simulink model "TargetPosVel"  (R2025a)
settings: Solver=ode4  StartTime=0.0  StopTime=stopTime  FixedStep=timeStep  RelTol=1e-3
values from neighbouring files (symbols this model uses):
  rand_vec = [0, rand(), rand()]    [model_parameters.m]
undefined symbols (not defined in the file or in its folder): angular_rate_noise_ON, angular_rate_noise_power, c, CD, dayValue, dimx, dimz, hourValue, I, I_W, IAU, K_optics, kd, kq, max_h, max_t, minuteValue, mu_E, Omega_E, Phi, pointing_body, q, quat0, quaternion_bias, quaternion_noise_ON, quaternion_sigma, R_E, rcp, res_dipole, secondValue, sma, timeStep, w0, WMM2020, yearValue
libraries: aerolibutil x19, matrix_library x10, aerolibtransform2 x8, vrlib x5, simulink x1, sharedTrackingLibrary x1, aerolibatmos2 x1, aerolibgravity2 x1, sharedtransform x1, sensorgpslib x1, visionsources x1
(part 1 of 2)
settings Model: Creator=nicolasgagliardi  LastModifiedBy=ako

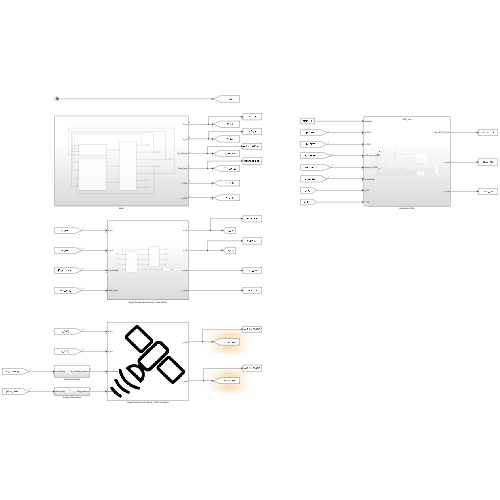
[thumbnail: Simulink's stored preview of the top-level diagram]
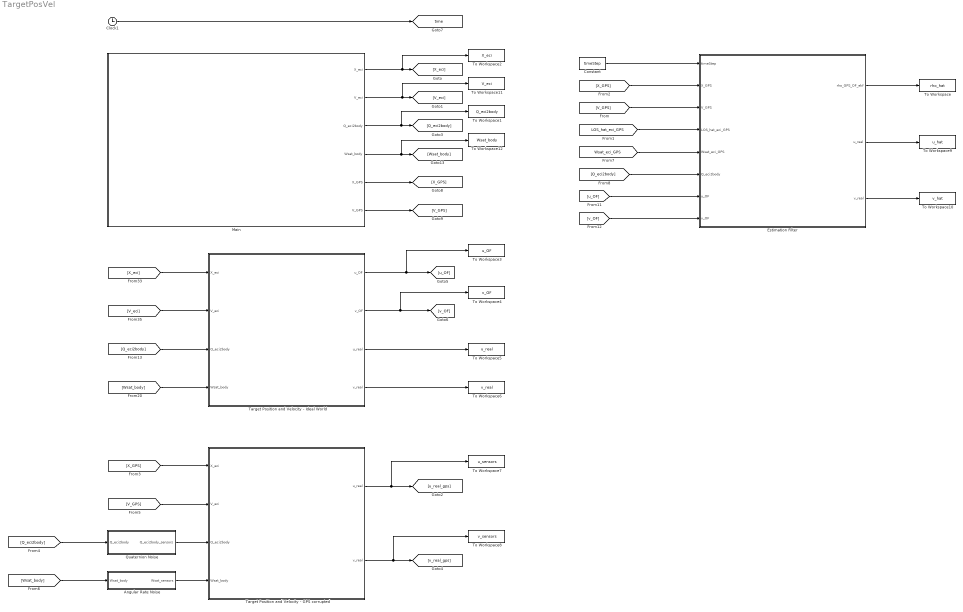
== system TargetPosVel ==
  Angular Rate Noise : Subsystem
  Clock1 : Clock
  Constant : Constant  Value=timeStep
  Estimation Filter : Subsystem  Variant=on  EmptyChoice=on
  Main : Subsystem
  Quaternion Noise : Subsystem
  Target Position and Velocity - GPS corrupted : Subsystem
      mask Display: image('gps.png');
  Target Position and Velocity - Ideal World : Subsystem
  To Workspace : ToWorkspace  VariableName=rho_hat  SaveFormat=Timeseries  SampleTime=-1
  To Workspace1 : ToWorkspace  VariableName=Q_eci2body  SaveFormat=Timeseries  SampleTime=-1
  To Workspace10 : ToWorkspace  VariableName=v_hat  SaveFormat=Timeseries  SampleTime=-1
  To Workspace11 : ToWorkspace  VariableName=V_eci  SaveFormat=Timeseries  SampleTime=-1
  To Workspace12 : ToWorkspace  VariableName=Wsat_body  SaveFormat=Timeseries  SampleTime=-1
  To Workspace2 : ToWorkspace  VariableName=X_eci  SaveFormat=Timeseries  SampleTime=-1
  To Workspace3 : ToWorkspace  VariableName=u_OF  SaveFormat=Timeseries  SampleTime=-1
  To Workspace4 : ToWorkspace  VariableName=v_OF  SaveFormat=Timeseries  SampleTime=-1
  To Workspace5 : ToWorkspace  VariableName=u_real  SaveFormat=Timeseries  SampleTime=-1
  To Workspace6 : ToWorkspace  VariableName=v_real  SaveFormat=Timeseries  SampleTime=-1
  To Workspace7 : ToWorkspace  VariableName=u_sensors  SaveFormat=Timeseries  SampleTime=-1
  To Workspace8 : ToWorkspace  VariableName=v_sensors  SaveFormat=Timeseries  SampleTime=-1
  To Workspace9 : ToWorkspace  VariableName=u_hat  SaveFormat=Timeseries  SampleTime=-1
  tag scope: time=global
  wires:
  [Q_eci2body] -> Target Position and Velocity - Ideal World/3(Q_eci2body)
  [Wsat_body] -> Target Position and Velocity - Ideal World/4(Wsat_body)
  Main/1(X_eci) -> [X_eci], To Workspace2/1
  Main/3(Q_eci2body) -> [Q_eci2body], To Workspace1/1
  Main/4(Wsat_body) -> To Workspace12/1, [Wsat_body]
  Main/2(V_eci) -> [V_eci], To Workspace11/1
  Target Position and Velocity - Ideal World/1(u_OF) -> To Workspace3/1, [u_OF]
  Main/5(X_GPS) -> [X_GPS]
  Main/6(V_GPS) -> [V_GPS]
  [V_eci] -> Target Position and Velocity - Ideal World/2(V_eci)
  Target Position and Velocity - GPS corrupted/1(u_real) -> [u_real_gps], To Workspace7/1
  Target Position and Velocity - GPS corrupted/2(v_real) -> [v_real_gps], To Workspace8/1
  [X_eci] -> Target Position and Velocity - Ideal World/1(X_eci)
  [X_GPS] -> Target Position and Velocity - GPS corrupted/1(X_eci)
  [V_GPS] -> Target Position and Velocity - GPS corrupted/2(V_eci)
  Target Position and Velocity - Ideal World/4(v_real) -> To Workspace6/1
  Target Position and Velocity - Ideal World/3(u_real) -> To Workspace5/1
  [Wsat_body] -> Angular Rate Noise/1(Wsat_body)
  Target Position and Velocity - Ideal World/2(v_OF) -> [v_OF], To Workspace4/1
  Clock1/1 -> [time]
  [Q_eci2body] -> Quaternion Noise/1(Q_eci2body)
  Quaternion Noise/1(Q_eci2body_sensors) -> Target Position and Velocity - GPS corrupted/3(Q_eci2body)
  Angular Rate Noise/1(Wsat_sensors) -> Target Position and Velocity - GPS corrupted/4(Wsat_body)
  Constant/1 -> Estimation Filter/1(timeStep)
  [X_GPS] -> Estimation Filter/2(X_GPS)
  [V_GPS] -> Estimation Filter/3(V_GPS)
  [LOS_hat_eci_GPS] -> Estimation Filter/4(LOS_hat_eci_GPS)
  [Wsat_eci_GPS] -> Estimation Filter/5(Wsat_eci_GPS)
  [Q_eci2body] -> Estimation Filter/6(Q_eci2body)
  [u_OF] -> Estimation Filter/7(u_OF)
  [v_OF] -> Estimation Filter/8(v_OF)
  Estimation Filter/1(rho_GPS_OF_ekf) -> To Workspace/1
  Estimation Filter/2(u_real) -> To Workspace9/1
  Estimation Filter/3(v_real) -> To Workspace10/1

== system TargetPosVel/Angular Rate Noise ==
  Wsat_body : Inport
  Add : Sum
  Band-Limited White Noise : simulink/Sources/Band-Limited White Noise  Cov=[angular_rate_noise_power]  Ts=timeStep  seed=[23341,23342,23343]
  Constant : Constant  Value=angular_rate_noise_ON
  Switch : Switch  Criteria=u2 ~= 0  SaturateOnIntegerOverflow=off  InputSameDT=off
  Wsat_sensors : Outport
  wires:
  Wsat_body/1 -> Switch/3, Add/2
  Add/1 -> Switch/1
  Constant/1 -> Switch/2
  Switch/1 -> Wsat_sensors/1
  Band-Limited White Noise/1 -> Add/1

== system TargetPosVel/Estimation Filter ==
  timeStep : Inport
  X_GPS : Inport  Port=2
  V_GPS : Inport  Port=3
  LOS_hat_eci_GPS : Inport  Port=4
  Wsat_eci_GPS : Inport  Port=5
  Q_eci2body : Inport  Port=6
  u_OF : Inport  Port=7
  v_OF : Inport  Port=8
  EKF_rho : Subsystem  VariantControl="estimation_filter == \"EKF_rho\""
  rho_GPS_OF_ekf : Outport
  u_real : Outport  Port=2
  v_real : Outport  Port=3

== system TargetPosVel/Main ==
  Attiude Controller : Subsystem  Variant=on  EmptyChoice=on
  Environmental Torques : Subsystem  Variant=on  EmptyChoice=on
  Spacecraft Dynamics : Subsystem
  X_eci : Outport
  V_eci : Outport  Port=2
  Q_eci2body : Outport  Port=3
  Wsat_body : Outport  Port=4
  X_GPS : Outport  Port=5
  V_GPS : Outport  Port=6
  wires:
  Spacecraft Dynamics/1(X_eci) -> Attiude Controller/1(r_ECI), Environmental Torques/1(X_eci), X_eci/1
  Spacecraft Dynamics/2(V_eci) -> Environmental Torques/2(V_eci), Attiude Controller/2(v_ECI), V_eci/1
  Spacecraft Dynamics/3(Q_eci2body) -> Environmental Torques/3(qECI2body), Attiude Controller/4(q_ECI2body), Q_eci2body/1
  Spacecraft Dynamics/4(W_sat_body) -> Attiude Controller/3(omega_b), Wsat_body/1
  Spacecraft Dynamics/6(X_GPS) -> X_GPS/1
  Spacecraft Dynamics/7(V_GPS) -> V_GPS/1
  Attiude Controller/1(h) -> Spacecraft Dynamics/2(h_rw)
  Attiude Controller/2(dh_dt) -> Spacecraft Dynamics/3(hdot_rw)
  Spacecraft Dynamics/5(t_JD) -> Environmental Torques/4(t_JD)
  Environmental Torques/1(T_env) -> Spacecraft Dynamics/1(T_env)

== system TargetPosVel/Quaternion Noise ==
  Q_eci2body : Inport
  Constant : Constant  Value=quaternion_noise_ON
  Constant1 : Constant  Value=quaternion_bias
  Constant2 : Constant  Value=quaternion_sigma
  MATLAB Function : MATLAB Function  TreatAsAtomicUnit=on
  Quaternion Multiplication : aerolibutil/Quaternion Multiplication
  Quaternion Multiplication2 : aerolibutil/Quaternion Multiplication
  Rotation Angles to Quaternions : Angle2Quat
      settings: AttributesFormatString=Rotation Order: %<rotationOrder>
  Rotation Angles to Quaternions1 : Angle2Quat
      settings: AttributesFormatString=Rotation Order: %<rotationOrder>
  Signal Specification : SignalSpecification  Dimensions=3
  Switch : Switch  Criteria=u2 ~= 0  SaturateOnIntegerOverflow=off  InputSameDT=off
  Q_eci2body_sensors : Outport
  wires:
  Q_eci2body/1 -> Quaternion Multiplication/2, Switch/3
  Rotation Angles to Quaternions/1 -> Quaternion Multiplication/1
  Switch/1 -> Q_eci2body_sensors/1
  Constant/1 -> Switch/2
  Constant1/1 -> Rotation Angles to Quaternions/1
  Constant2/1 -> MATLAB Function/1(quaternion_sigma)
  MATLAB Function/1(angle_noise) -> Signal Specification/1
  Quaternion Multiplication/1 -> Quaternion Multiplication2/2
  Quaternion Multiplication2/1 -> Switch/1
  Signal Specification/1 -> Rotation Angles to Quaternions1/1
  Rotation Angles to Quaternions1/1 -> Quaternion Multiplication2/1

== system TargetPosVel/Target Position and Velocity - GPS corrupted ==
  X_eci : Inport
  V_eci : Inport  Port=2
  Q_eci2body : Inport  Port=3
  Wsat_body : Inport  Port=4
  LLA conversion : Subsystem
  LOS Calculations : Subsystem
  Pixel shift : Subsystem
  To Workspace : ToWorkspace  VariableName=lla_tar_gps  SampleTime=-1
  u_real : Outport
  v_real : Outport  Port=2
  wires:
  LOS Calculations/3(Vtar_eci) -> Pixel shift/4(Vtar_eci)
  LOS Calculations/2(Rtar_eci) -> Pixel shift/3(Rtar_eci)
  LLA conversion/1(LLAtar) -> To Workspace/1
  LOS Calculations/4(Rtar_ecef) -> LLA conversion/1(Rtar_ecef)
  LOS Calculations/1(rho) -> Pixel shift/2(rho)
  Pixel shift/2(v_real) -> v_real/1
  Pixel shift/1(u_real) -> u_real/1
  Wsat_body/1 -> LOS Calculations/4(Wsat_b)
  X_eci/1 -> LOS Calculations/3(Rsat)
  V_eci/1 -> LOS Calculations/2(Vsat)
  Q_eci2body/1 -> LOS Calculations/1(Q_eci2body), Pixel shift/1(Q_eci2body)

== system TargetPosVel/Target Position and Velocity - Ideal World ==
  X_eci : Inport
  V_eci : Inport  Port=2
  Q_eci2body : Inport  Port=3
  Wsat_body : Inport  Port=4
  LLA conversion : Subsystem
  LOS Calculations : Subsystem
  Pixel shift : Subsystem
  To Workspace : ToWorkspace  VariableName=lla_tar  SampleTime=-1
  u_OF : Outport
  v_OF : Outport  Port=2
  u_real : Outport  Port=3
  v_real : Outport  Port=4
  wires:
  Q_eci2body/1 -> LOS Calculations/1(Q_eci2body), Pixel shift/1(Q_eci2body)
  V_eci/1 -> LOS Calculations/2(Vsat)
  X_eci/1 -> LOS Calculations/3(Rsat)
  Wsat_body/1 -> LOS Calculations/4(Wsat_b)
  Pixel shift/1(u_OF) -> u_OF/1
  Pixel shift/2(v_OF) -> v_OF/1
  LOS Calculations/1(rho) -> Pixel shift/2(rho)
  LOS Calculations/4(Rtar_ecef) -> LLA conversion/1(Rtar_ecef)
  LLA conversion/1(LLAtar) -> To Workspace/1
  LOS Calculations/2(Rtar_eci) -> Pixel shift/3(Rtar_eci)
  LOS Calculations/3(Vtar_eci) -> Pixel shift/4(Vtar_eci)
  Pixel shift/3(u_real) -> u_real/1
  Pixel shift/4(v_real) -> v_real/1

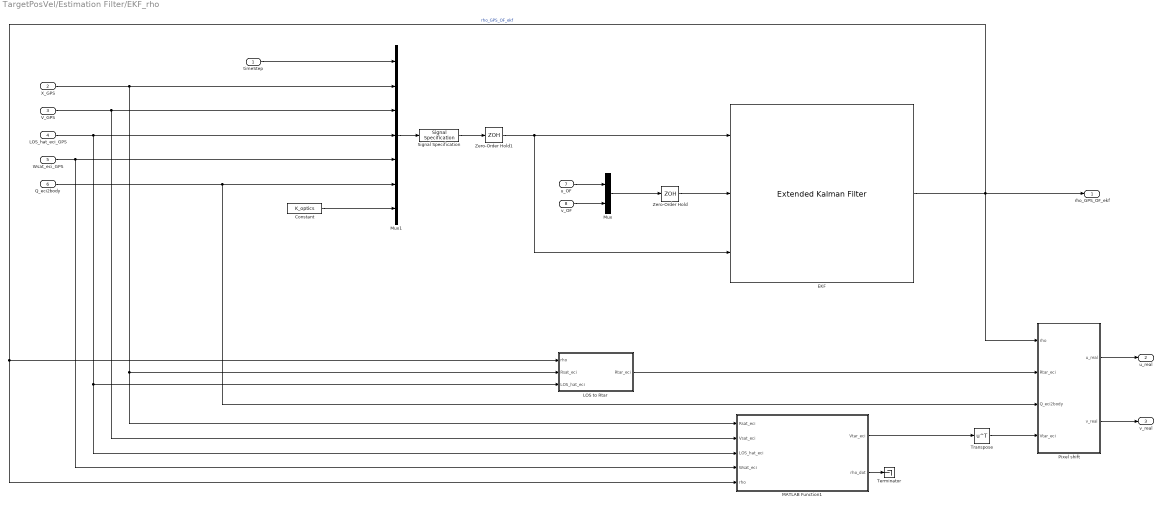
== system TargetPosVel/Estimation Filter/EKF_rho ==
  timeStep : Inport
  X_GPS : Inport  Port=2
  V_GPS : Inport  Port=3
  LOS_hat_eci_GPS : Inport  Port=4
  Wsat_eci_GPS : Inport  Port=5
  Q_eci2body : Inport  Port=6
  u_OF : Inport  Port=7
  v_OF : Inport  Port=8
  Constant : Constant  Value=K_optics
  EKF : sharedTrackingLibrary/Extended Kalman Filter  StateTransitionFcn=rhoSTF  HasStateTransitionJacobianFcn=off  HasAdditiveProcessNoise=Additive  ProcessNoise=Q  HasTimeVaryingProcessNoise=off  HasStateTransitionFcnExtraArgument=1  InitialState=rho_0  InitialStateCovariance=20  MeasurementFcn1=rhoMF  HasMeasurementJacobianFcn1=off  HasMeasurementEnablePort1=off  HasAdditiveMeasurementNoise1=Additive  MeasurementNoise1=[0.1,0;0,0.1]  HasTimeVaryingMeasurementNoise1=off  HasMeasurementFcnExtraArgument1=1  HasMeasurementWrapping1=off  MeasurementFcn2=myMeasurementFcn  HasMeasurementJacobianFcn2=off  HasMeasurementEnablePort2=off  HasAdditiveMeasurementNoise2=Additive  MeasurementNoise2=1  HasTimeVaryingMeasurementNoise2=off  HasMeasurementFcnExtraArgument2=0  HasMeasurementWrapping2=off  MeasurementFcn3=myMeasurementFcn  HasMeasurementJacobianFcn3=off  HasMeasurementEnablePort3=off  HasAdditiveMeasurementNoise3=Additive  MeasurementNoise3=1  HasTimeVaryingMeasurementNoise3=off  HasMeasurementFcnExtraArgument3=0  HasMeasurementWrapping3=off  MeasurementFcn4=myMeasurementFcn  HasMeasurementJacobianFcn4=off  HasMeasurementEnablePort4=off  HasAdditiveMeasurementNoise4=Additive  MeasurementNoise4=1  HasTimeVaryingMeasurementNoise4=off  HasMeasurementFcnExtraArgument4=0  HasMeasurementWrapping4=off  MeasurementFcn5=myMeasurementFcn  HasMeasurementJacobianFcn5=off  HasMeasurementEnablePort5=off  HasAdditiveMeasurementNoise5=Additive  MeasurementNoise5=1  HasTimeVaryingMeasurementNoise5=off  HasMeasurementFcnExtraArgument5=0  HasMeasurementWrapping5=off  EnableMultirate=off  StateTransitionFcnSampleTime=1  MeasurementFcn1SampleTime=1  MeasurementFcn2SampleTime=1  MeasurementFcn3SampleTime=1  MeasurementFcn4SampleTime=1  MeasurementFcn5SampleTime=1  UseCurrentEstimator=on  OutputStateCovariance=off  DataType=double  SampleTime=timeStep  NumberOfMeasurements=1
  LOS to Rtar : Subsystem
  MATLAB Function1 : MATLAB Function  TreatAsAtomicUnit=on
  Mux : Mux  Inputs=2
  Mux1 : Mux  Inputs=7
  Pixel shift : Subsystem
  Signal Specification : SignalSpecification  Dimensions=18
  Terminator : Terminator
  Transpose : Math  Operator=transpose
  Zero-Order Hold : ZeroOrderHold  SampleTime=timeStep
  Zero-Order Hold1 : ZeroOrderHold  SampleTime=timeStep
  rho_GPS_OF_ekf : Outport
  u_real : Outport  Port=2
  v_real : Outport  Port=3
  wires:
  timeStep/1 -> Mux1/1
  Mux1/1 -> Signal Specification/1
  Q_eci2body/1 -> Mux1/6, Pixel shift/3(Q_eci2body)
  Zero-Order Hold/1 -> EKF/2
  Zero-Order Hold1/1 -> EKF/1, EKF/3
  Mux/1 -> Zero-Order Hold/1
  Signal Specification/1 -> Zero-Order Hold1/1
  Wsat_eci_GPS/1 -> Mux1/5, MATLAB Function1/4(Wsat_eci)
  v_OF/1 -> Mux/2
  X_GPS/1 -> Mux1/2, MATLAB Function1/1(Rsat_eci), LOS to Rtar/2(Rsat_eci)
  LOS_hat_eci_GPS/1 -> Mux1/4, MATLAB Function1/3(LOS_hat_eci), LOS to Rtar/3(LOS_hat_eci)
  V_GPS/1 -> Mux1/3, MATLAB Function1/2(Vsat_eci)
  u_OF/1 -> Mux/1
  EKF/1 -> Pixel shift/1(rho), MATLAB Function1/5(rho), LOS to Rtar/1(rho), rho_GPS_OF_ekf/1  "rho_GPS_OF_ekf"
  Pixel shift/2(v_real) -> v_real/1
  Pixel shift/1(u_real) -> u_real/1
  MATLAB Function1/2(rho_dot) -> Terminator/1
  Constant/1 -> Mux1/7
  MATLAB Function1/1(Vtar_eci) -> Transpose/1
  Transpose/1 -> Pixel shift/4(Vtar_eci)
  LOS to Rtar/1(Rtar_eci) -> Pixel shift/2(Rtar_eci)

== system TargetPosVel/Main/Attiude Controller ==
  r_ECI : Inport
  v_ECI : Inport  Port=2
  omega_b : Inport  Port=3
  q_ECI2body : Inport  Port=4
  Controller OFF : Subsystem  VariantControl=controller_ON == 0
  Nadir Pointing Controller : Subsystem  VariantControl=controller_ON == 1
  h : Outport
  dh_dt : Outport  Port=2

== system TargetPosVel/Main/Environmental Torques ==
  X_eci : Inport
  V_eci : Inport  Port=2
  qECI2body : Inport  Port=3
  t_JD : Inport  Port=4
  Environmental Torques : Subsystem  VariantControl=env_torques_ON == 1
  Environmental Torques OFF : Subsystem  VariantControl=env_torques_ON == 0
  T_env : Outport

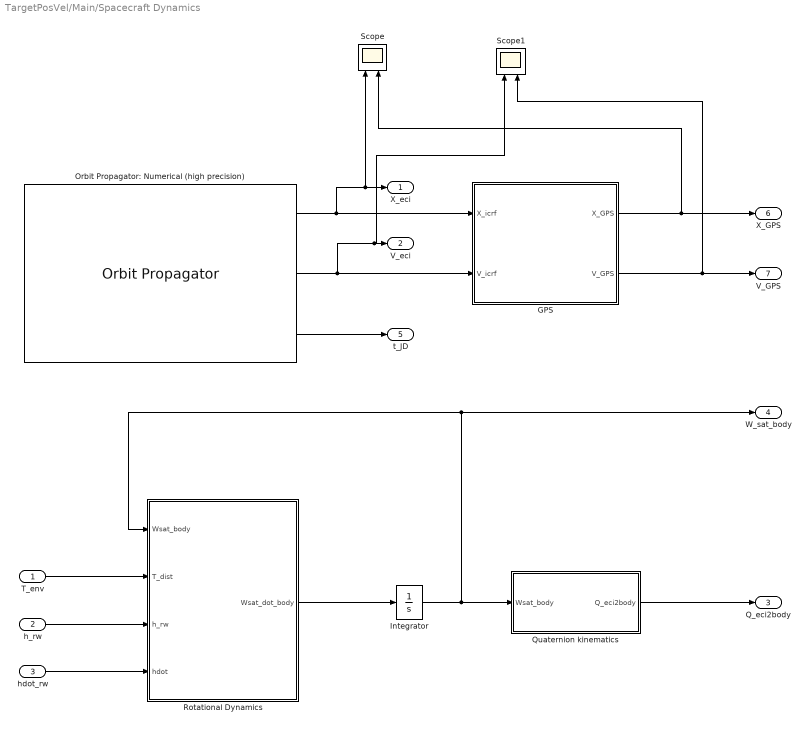
== system TargetPosVel/Main/Spacecraft Dynamics ==
  T_env : Inport
  h_rw : Inport  Port=2
  hdot_rw : Inport  Port=3
  GPS : Subsystem
  Integrator : Integrator  InitialCondition=w0
  Orbit Propagator: Numerical (high precision) : OrbitPropagator  propagator=Numerical (high precision)  startDate=jdate  mass=mass  action=None  semiMajorAxis=sma  eccentricity=ecc  inclination=inc_SSO  raan=RAAN  argPeriapsis=aop  trueAnomaly=truean  inertialPosition=[3649700.0 3308200.0 -4676600.0]  inertialVelocity=[-2750.8 6666.4 2573.4]  fixedPosition=[-4142689.0 -2676864.7 -4669861.6]  fixedVelocity=[1452.7 -6720.7 2568.1]  customR=3396200  customMu=4.305e13  customJ2=1.0826269e-03  customOmega=4.06125949e-3  F107ExtrapMethod=Least squares fit  MagneticIndexExtrapMethod=IGRF  dragCoeff=CD  dragArea=dimx*dimz  useEphemerisDateRange=off  ephemerisStartDate=jdate  ephemerisEndDate=jdate  includeSunGravity=off  reflectivityCoeff=q  srpArea=dimx*dimz
  Quaternion kinematics : Subsystem
  Rotational Dynamics : Subsystem
  Scope : Scope  NumInputPorts=2
      settings: ActiveDisplayYMinimum=-12780.9796153992  ActiveDisplayYMaximum=52179.154390941323
  Scope1 : Scope  NumInputPorts=2
      settings: ActiveDisplayYMinimum=-40.67155384373234  ActiveDisplayYMaximum=0.53047510275488818  DataLoggingVariableName=ScopeData4
  X_eci : Outport
  V_eci : Outport  Port=2
  Q_eci2body : Outport  Port=3
  W_sat_body : Outport  Port=4
  t_JD : Outport  Port=5
  X_GPS : Outport  Port=6
  V_GPS : Outport  Port=7
  wires:
  Orbit Propagator: Numerical (high precision)/3 -> t_JD/1
  Integrator/1 -> Quaternion kinematics/1(Wsat_body), W_sat_body/1, Rotational Dynamics/1(Wsat_body)
  GPS/1(X_GPS) -> X_GPS/1, Scope/2
  GPS/2(V_GPS) -> V_GPS/1, Scope1/2
  Orbit Propagator: Numerical (high precision)/1 -> GPS/1(X_icrf), X_eci/1, Scope/1
  T_env/1 -> Rotational Dynamics/2(T_dist)
  Rotational Dynamics/1(Wsat_dot_body) -> Integrator/1
  h_rw/1 -> Rotational Dynamics/3(h_rw)
  Orbit Propagator: Numerical (high precision)/2 -> Scope1/1, V_eci/1, GPS/2(V_icrf)
  hdot_rw/1 -> Rotational Dynamics/4(hdot)
  Quaternion kinematics/1(Q_eci2body) -> Q_eci2body/1

== system TargetPosVel/Target Position and Velocity - GPS corrupted/LLA conversion ==
  Rtar_ecef : Inport
  ECEF Position to LLA : ECEF2LLA
  Mux : Mux  Inputs=2
  LLAtar : Outport
  wires:
  Mux/1 -> LLAtar/1
  ECEF Position to LLA/2 -> Mux/2
  ECEF Position to LLA/1 -> Mux/1
  Rtar_ecef/1 -> ECEF Position to LLA/1

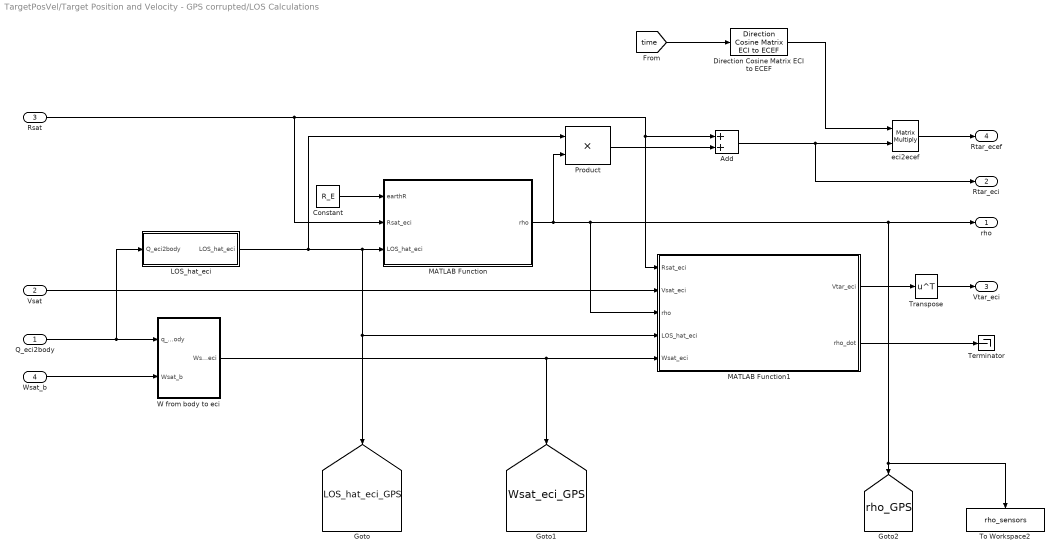
== system TargetPosVel/Target Position and Velocity - GPS corrupted/LOS Calculations ==
  Q_eci2body : Inport
  Vsat : Inport  Port=2
  Rsat : Inport  Port=3
  Wsat_b : Inport  Port=4
  Add : Sum
  Constant : Constant  Value=R_E
  Direction Cosine Matrix ECI to ECEF : aerolibtransform2/Direction Cosine Matrix ECI to ECEF  red=IAU-2000/2006  year=yearValue  month=January  day=1  hour=hourValue  min=minuteValue  sec=secondValue  deltaT=Sec  errorflag=Error  extraparamflag=off
      settings: AttributesFormatString=%<red>
  LOS_hat_eci : Subsystem
  MATLAB Function : MATLAB Function  TreatAsAtomicUnit=on
  MATLAB Function1 : MATLAB Function  TreatAsAtomicUnit=on
  Product : Product
  Terminator : Terminator
  To Workspace2 : ToWorkspace  VariableName=rho_sensors  SaveFormat=Timeseries  SampleTime=-1
  Transpose : Math  Operator=transpose
  "W from body to eci " : Subsystem
  eci2ecef : Product  Multiplication=Matrix(*)
  rho : Outport
  Rtar_eci : Outport  Port=2
  Vtar_eci : Outport  Port=3
  Rtar_ecef : Outport  Port=4
  tag scope: LOS_hat_eci_GPS=global, Wsat_eci_GPS=global, rho_GPS=global
  wires:
  eci2ecef/1 -> Rtar_ecef/1
  Add/1 -> Rtar_eci/1, eci2ecef/2
  Direction Cosine Matrix ECI to ECEF/1 -> eci2ecef/1
  Vsat/1 -> MATLAB Function1/2(Vsat_eci)
  LOS_hat_eci/1(LOS_hat_eci) -> Product/1, MATLAB Function/3(LOS_hat_eci), MATLAB Function1/4(LOS_hat_eci), [LOS_hat_eci_GPS]
  "W from body to eci "/1(Wsat_eci) -> [Wsat_eci_GPS], MATLAB Function1/5(Wsat_eci)
  Constant/1 -> MATLAB Function/1(earthR)
  Wsat_b/1 -> "W from body to eci "/2(Wsat_b)
  Rsat/1 -> MATLAB Function/2(Rsat_eci), Add/1, MATLAB Function1/1(Rsat_eci)
  MATLAB Function/1(rho) -> Product/2, MATLAB Function1/3(rho), rho/1, To Workspace2/1, [rho_GPS]
  Q_eci2body/1 -> "W from body to eci "/1(q_eci2body), LOS_hat_eci/1(Q_eci2body)
  Product/1 -> Add/2
  MATLAB Function1/2(rho_dot) -> Terminator/1
  MATLAB Function1/1(Vtar_eci) -> Transpose/1
  Transpose/1 -> Vtar_eci/1
  [time] -> Direction Cosine Matrix ECI to ECEF/1

== system TargetPosVel/Target Position and Velocity - GPS corrupted/Pixel shift ==
  Q_eci2body : Inport
  rho : Inport  Port=2
  Rtar_eci : Inport  Port=3
  Vtar_eci : Inport  Port=4
  Constant : Constant  Value=[0;0;Omega_E]
  Selector2 : Selector  InputPortWidth=3  IndexOptions=Index vector (dialog)  Indices=[1 2]  OutputSizes=1
  UV calculation : Subsystem
  Vim_body : Subsystem
  Vim_eci : Subsystem
  u_real : Outport
  v_real : Outport  Port=2
  wires:
  Constant/1 -> Vim_eci/3(We_eci)
  UV calculation/2(v_real) -> v_real/1
  UV calculation/1(u_real) -> u_real/1
  Vim_eci/1(Vim_eci) -> Vim_body/2(vec)
  Vim_body/1(vec_rot) -> Selector2/1
  rho/1 -> UV calculation/2(rho)
  Vtar_eci/1 -> Vim_eci/2(Vtar_eci)
  Q_eci2body/1 -> Vim_body/1(q)
  Selector2/1 -> UV calculation/1(Vim_body)
  Rtar_eci/1 -> Vim_eci/1(Rtar_eci)

== system TargetPosVel/Target Position and Velocity - Ideal World/LLA conversion ==
  Rtar_ecef : Inport
  ECEF Position to LLA : ECEF2LLA
  Mux : Mux  Inputs=2
  LLAtar : Outport
  wires:
  Rtar_ecef/1 -> ECEF Position to LLA/1
  ECEF Position to LLA/1 -> Mux/1
  ECEF Position to LLA/2 -> Mux/2
  Mux/1 -> LLAtar/1

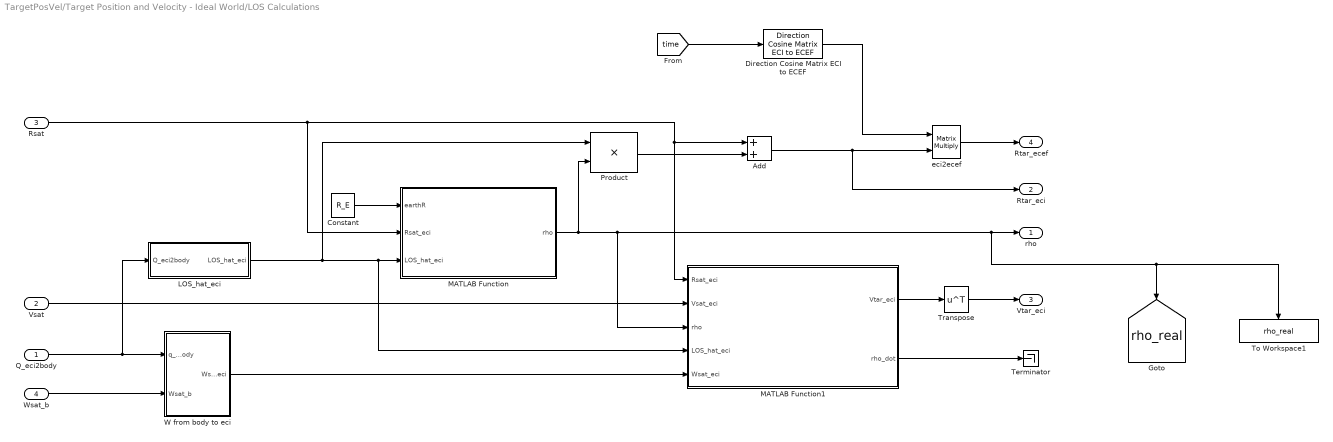
== system TargetPosVel/Target Position and Velocity - Ideal World/LOS Calculations ==
  Q_eci2body : Inport
  Vsat : Inport  Port=2
  Rsat : Inport  Port=3
  Wsat_b : Inport  Port=4
  Add : Sum
  Constant : Constant  Value=R_E
  Direction Cosine Matrix ECI to ECEF : aerolibtransform2/Direction Cosine Matrix ECI to ECEF  red=IAU-2000/2006  year=yearValue  month=January  day=1  hour=hourValue  min=minuteValue  sec=secondValue  deltaT=Sec  errorflag=Error  extraparamflag=off
      settings: AttributesFormatString=%<red>
  LOS_hat_eci : Subsystem
  MATLAB Function : MATLAB Function  TreatAsAtomicUnit=on
  MATLAB Function1 : MATLAB Function  TreatAsAtomicUnit=on
  Product : Product
  Terminator : Terminator
  To Workspace1 : ToWorkspace  VariableName=rho_real  SaveFormat=Timeseries  SampleTime=-1
  Transpose : Math  Operator=transpose
  "W from body to eci " : Subsystem
  eci2ecef : Product  Multiplication=Matrix(*)
  rho : Outport
  Rtar_eci : Outport  Port=2
  Vtar_eci : Outport  Port=3
  Rtar_ecef : Outport  Port=4
  tag scope: rho_real=global
  wires:
  Product/1 -> Add/2
  Q_eci2body/1 -> LOS_hat_eci/1(Q_eci2body), "W from body to eci "/1(q_eci2body)
  MATLAB Function/1(rho) -> [rho_real], To Workspace1/1, rho/1, MATLAB Function1/3(rho), Product/2
  Rsat/1 -> MATLAB Function1/1(Rsat_eci), Add/1, MATLAB Function/2(Rsat_eci)
  Wsat_b/1 -> "W from body to eci "/2(Wsat_b)
  Constant/1 -> MATLAB Function/1(earthR)
  "W from body to eci "/1(Wsat_eci) -> MATLAB Function1/5(Wsat_eci)
  LOS_hat_eci/1(LOS_hat_eci) -> MATLAB Function1/4(LOS_hat_eci), MATLAB Function/3(LOS_hat_eci), Product/1
  Vsat/1 -> MATLAB Function1/2(Vsat_eci)
  Direction Cosine Matrix ECI to ECEF/1 -> eci2ecef/1
  Add/1 -> eci2ecef/2, Rtar_eci/1
  eci2ecef/1 -> Rtar_ecef/1
  MATLAB Function1/2(rho_dot) -> Terminator/1
  MATLAB Function1/1(Vtar_eci) -> Transpose/1
  Transpose/1 -> Vtar_eci/1
  [time] -> Direction Cosine Matrix ECI to ECEF/1

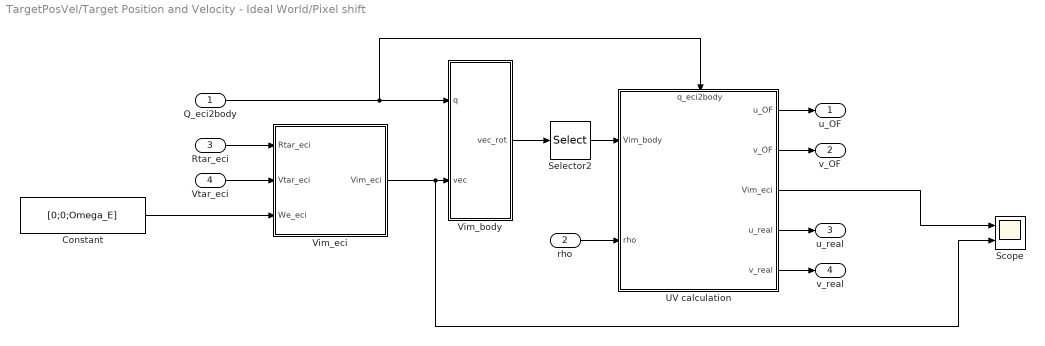
== system TargetPosVel/Target Position and Velocity - Ideal World/Pixel shift ==
  Q_eci2body : Inport
  rho : Inport  Port=2
  Rtar_eci : Inport  Port=3
  Vtar_eci : Inport  Port=4
  Constant : Constant  Value=[0;0;Omega_E]
  Scope : Scope  NumInputPorts=2
      settings: ActiveDisplayYMinimum=7345.085472920141  ActiveDisplayYMaximum=7801.8686248677177  DataLoggingVariableName=ScopeData5
  Selector2 : Selector  InputPortWidth=3  IndexOptions=Index vector (dialog)  Indices=[1 2]  OutputSizes=1
  UV calculation : Subsystem
      settings: PortSchema="{\"entries\":[{\"content\":{\"sides\":[{\"content\":{\"connectorIds\":[\"In1\",\"In2\"]},\"type\":\"ConnectorPlacement.EquallySpacedRectSide\",\"uuid\":\"7d962072-08bb-43f9-8096-b084f9aeb233\"},{\"content\":{\"connectorIds\":[\"Out1\",\"Out2\",\"Out3\",\"Out4\",\"Out5\"],\"side\":\"RIGHT\"},\"type\":\"ConnectorPlacement.EquallySpacedRectSide\",\"uuid\":\"b4a50fa6-2234-460e-9b12-c6b5a2f30818\"},{\"content\":{\"connectorIds\":[\"In3\"],\"side\":\"TOP\"},\"type\":\"ConnectorPlacement.EquallySpacedRectSide\",\"uuid\":\"25b05795-271b-402f-b612-88591474e4ef\"}]},\"type\":\"ConnectorPlacement.EquallySpacedConnector\",\"uuid\":\"2e7139ee-cebd-46fb-9053-110263a5a01d\"}],\"packageUris\":[\"http://schema.mathworks.com/mf0/Connector/R2020b\"],\"version\":\"1.0\"}"
  Vim_body : Subsystem
  Vim_eci : Subsystem
  u_OF : Outport
  v_OF : Outport  Port=2
  u_real : Outport  Port=3
  v_real : Outport  Port=4
  wires:
  Rtar_eci/1 -> Vim_eci/1(Rtar_eci)
  Selector2/1 -> UV calculation/1(Vim_body)
  Q_eci2body/1 -> Vim_body/1(q), UV calculation/3(q_eci2body)
  Vtar_eci/1 -> Vim_eci/2(Vtar_eci)
  rho/1 -> UV calculation/2(rho)
  Vim_body/1(vec_rot) -> Selector2/1
  Vim_eci/1(Vim_eci) -> Scope/2, Vim_body/2(vec)
  UV calculation/1(u_OF) -> u_OF/1
  UV calculation/2(v_OF) -> v_OF/1
  Constant/1 -> Vim_eci/3(We_eci)
  UV calculation/3(Vim_eci) -> Scope/1
  UV calculation/4(u_real) -> u_real/1
  UV calculation/5(v_real) -> v_real/1

== system TargetPosVel/Estimation Filter/EKF_rho/LOS to Rtar ==
  rho : Inport
  Rsat_eci : Inport  Port=2
  LOS_hat_eci : Inport  Port=3
  Add : Sum
  Product : Product
  Rtar_eci : Outport
  wires:
  LOS_hat_eci/1 -> Product/1
  rho/1 -> Product/2
  Product/1 -> Add/1
  Rsat_eci/1 -> Add/2
  Add/1 -> Rtar_eci/1

== system TargetPosVel/Estimation Filter/EKF_rho/Pixel shift ==
  rho : Inport
  Rtar_eci : Inport  Port=2
  Q_eci2body : Inport  Port=3
  Vtar_eci : Inport  Port=4
  Constant : Constant  Value=[0;0;Omega_E]
  Selector2 : Selector  InputPortWidth=3  IndexOptions=Index vector (dialog)  Indices=[1 2]  OutputSizes=1
  UV calculation : Subsystem
  Vim_body : Subsystem
  Vim_eci : Subsystem
  u_real : Outport
  v_real : Outport  Port=2
  wires:
  Constant/1 -> Vim_eci/3(We_eci)
  UV calculation/2(v_real) -> v_real/1
  UV calculation/1(u_real) -> u_real/1
  Vim_body/1(vec_rot) -> Selector2/1
  rho/1 -> UV calculation/2(rho)
  Vtar_eci/1 -> Vim_eci/2(Vtar_eci)
  Q_eci2body/1 -> Vim_body/1(q)
  Selector2/1 -> UV calculation/1(Vim_body)
  Rtar_eci/1 -> Vim_eci/1(Rtar_eci)
  Vim_eci/1(Vim_eci) -> Vim_body/2(vec)

== system TargetPosVel/Main/Attiude Controller/Controller OFF ==
  Constant : Constant  Value=0
  Constant1 : Constant  Value=0
  h : Outport
  dh_dt : Outport  Port=2
  wires:
  Constant/1 -> h/1
  Constant1/1 -> dh_dt/1

== system TargetPosVel/Main/Attiude Controller/Nadir Pointing Controller ==
  r_ECI : Inport
  v_ECI : Inport  Port=2
  omega_b : Inport  Port=3
  q_ECI2body : Inport  Port=4
  Nadir Pointing : Subsystem  TreatAsAtomicUnit=on
  Nadir pointing : Subsystem
  RW Saturation : Subsystem
  h : Outport
  dh_dt : Outport  Port=2
  wires:
  omega_b/1 -> Nadir pointing/2(omega_b), RW Saturation/2(omega)
  RW Saturation/2(dh_dt) -> dh_dt/1
  RW Saturation/1(h) -> h/1
  Nadir pointing/1(g) -> RW Saturation/1(g)
  Nadir Pointing/1(q_Err) -> Nadir pointing/1(qErr)
  Nadir Pointing/2(w_des) -> Nadir pointing/3(omega_des_b)
  r_ECI/1 -> Nadir Pointing/1(r_ECI)
  v_ECI/1 -> Nadir Pointing/2(v_ECI)
  q_ECI2body/1 -> Nadir Pointing/3(q_ECI2body)

== system TargetPosVel/Main/Environmental Torques/Environmental Torques ==
  X_eci : Inport
  V_eci : Inport  Port=2
  qECI2body : Inport  Port=3
  t_JD : Inport  Port=4
  Add : Sum  Inputs=++++
  "Aerodynamic Torque  " : Subsystem
  Gravity Gradient Torque : Subsystem
  Magnetic Torque : Subsystem
  Quaternions to Direction Cosine Matrix : sharedtransform/Quaternions to  Direction Cosine Matrix  aMode=aMode
  Solar Radiation Pressure Torque : Subsystem
  T_env : Outport
  wires:
  "Aerodynamic Torque  "/1(Tdrag) -> Add/2
  Quaternions to Direction Cosine Matrix/1 -> Magnetic Torque/2(DCM_eci2body), Solar Radiation Pressure Torque/1(DCM_eci2body), "Aerodynamic Torque  "/2(DCM_eci2body), Gravity Gradient Torque/1(DCM_eci2body)
  Gravity Gradient Torque/1(Tgg) -> Add/1
  X_eci/1 -> Solar Radiation Pressure Torque/2(X_eci), Magnetic Torque/1(X_eci), "Aerodynamic Torque  "/1(X_eci), Gravity Gradient Torque/2(X_eci)
  V_eci/1 -> "Aerodynamic Torque  "/3(V_eci)
  Solar Radiation Pressure Torque/1(T_srp) -> Add/3
  qECI2body/1 -> Quaternions to Direction Cosine Matrix/1
  t_JD/1 -> Solar Radiation Pressure Torque/3(t_JD)
  Magnetic Torque/1(Tmag) -> Add/4
  Add/1 -> T_env/1

== system TargetPosVel/Main/Environmental Torques/Environmental Torques OFF ==
  Constant : Constant  Value=0
  T_env : Outport
  wires:
  Constant/1 -> T_env/1

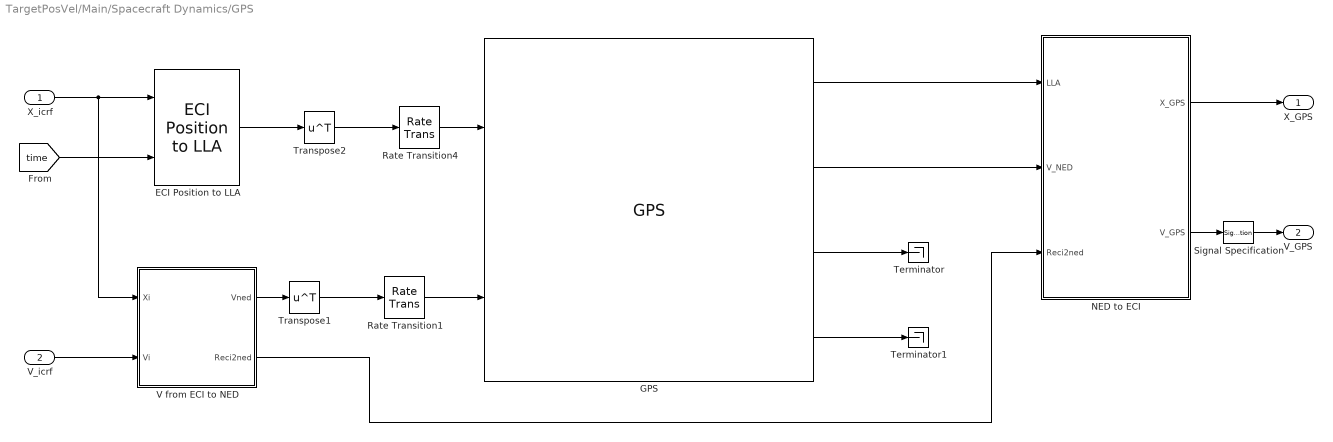
== system TargetPosVel/Main/Spacecraft Dynamics/GPS ==
  X_icrf : Inport
  V_icrf : Inport  Port=2
  ECI Position to LLA : aerolibtransform2/ECI Position to LLA  red=IAU-2000/2006  year=yearValue  month=January  day=1  hour=hourValue  min=minuteValue  sec=secondValue  deltaT=Sec  errorflag=Error  extraparamflag=off  eunits=Metric (MKS)  earthmodel=WGS84  flat=1/298.257223563  eqradius=6378137
      settings: AttributesFormatString=%<red>
  GPS : sensorgpslib/GPS  DispRefFrame=NED  PositionInputFormat=Geodetic  ReferenceLocation=[ 0, 0, 0 ]  HorizontalPositionAccuracy=GPSHAccuracy  VerticalPositionAccuracy=GPSVAccuracy  VelocityAccuracy=GPSVelAccuracy  DecayFactor=0  SeedDouble=67  SimulateUsing=Interpreted execution
  NED to ECI : Subsystem
  Rate Transition1 : RateTransition  OutPortSampleTime=timeStep
  Rate Transition4 : RateTransition  OutPortSampleTime=timeStep
  Signal Specification : SignalSpecification  Dimensions=3
  Terminator : Terminator
  Terminator1 : Terminator
  Transpose1 : Math  Operator=transpose
  Transpose2 : Math  Operator=transpose
  V from ECI to NED : Subsystem
  X_GPS : Outport
  V_GPS : Outport  Port=2
  wires:
  V_icrf/1 -> V from ECI to NED/2(Vi)
  ECI Position to LLA/1 -> Transpose2/1
  Rate Transition4/1 -> GPS/1
  Rate Transition1/1 -> GPS/2
  Transpose1/1 -> Rate Transition1/1
  Transpose2/1 -> Rate Transition4/1
  X_icrf/1 -> ECI Position to LLA/1, V from ECI to NED/1(Xi)
  GPS/3 -> Terminator/1
  GPS/4 -> Terminator1/1
  GPS/1 -> NED to ECI/1(LLA)
  GPS/2 -> NED to ECI/2(V_NED)
  NED to ECI/1(X_GPS) -> X_GPS/1
  V from ECI to NED/2(Reci2ned) -> NED to ECI/3(Reci2ned)
  V from ECI to NED/1(Vned) -> Transpose1/1
  [time] -> ECI Position to LLA/2
  Signal Specification/1 -> V_GPS/1
  NED to ECI/2(V_GPS) -> Signal Specification/1

== system TargetPosVel/Main/Spacecraft Dynamics/Quaternion kinematics ==
  Wsat_body : Inport
  Gain1 : Gain  Gain=0.5
  Integrator1 : Integrator  InitialCondition=quat0
  MATLAB Function : MATLAB Function  TreatAsAtomicUnit=on
  Product : Product  Multiplication=Matrix(*)
  Q_eci2body : Outport
  wires:
  Gain1/1 -> Product/1
  Wsat_body/1 -> MATLAB Function/1(omega)
  MATLAB Function/1(OMEGA) -> Gain1/1
  Integrator1/1 -> Q_eci2body/1, Product/2
  Product/1 -> Integrator1/1

== system TargetPosVel/Main/Spacecraft Dynamics/Rotational Dynamics ==
  Wsat_body : Inport
  T_dist : Inport  Port=2
  h_rw : Inport  Port=3
  hdot : Inport  Port=4
  Constant : Constant  Value=I
  Cross Product : matrix_library/Cross Product
  Invert 3x3 Matrix : aerolibutil/Invert  3x3 Matrix
  MatrixMultiply : Product  Multiplication=Matrix(*)
  MatrixMultiply1 : Product  Multiplication=Matrix(*)
  Minus : Sum  Inputs=+--
  Minus1 : Sum
  Wsat_dot_body : Outport
  wires:
  Invert 3x3 Matrix/1 -> MatrixMultiply1/1
  T_dist/1 -> Minus/1
  Minus1/1 -> Cross Product/2
  MatrixMultiply1/1 -> Wsat_dot_body/1
  Minus/1 -> MatrixMultiply1/2
  Constant/1 -> Invert 3x3 Matrix/1, MatrixMultiply/1
  Wsat_body/1 -> Cross Product/1, MatrixMultiply/2
  MatrixMultiply/1 -> Minus1/1
  Cross Product/1 -> Minus/2
  h_rw/1 -> Minus1/2
  hdot/1 -> Minus/3

== system TargetPosVel/Target Position and Velocity - GPS corrupted/LOS Calculations/LOS_hat_eci ==
  Q_eci2body : Inport
  Constant : Constant  Value=pointing_body
  Quaternion Inverse : aerolibutil/Quaternion Inverse
  Quaternion Rotation : aerolibutil/Quaternion Rotation
  LOS_hat_eci : Outport
  wires:
  Quaternion Rotation/1 -> LOS_hat_eci/1  "LOS_hat_eci"
  Constant/1 -> Quaternion Rotation/2
  Quaternion Inverse/1 -> Quaternion Rotation/1  "q_body2eci"
  Q_eci2body/1 -> Quaternion Inverse/1

== system TargetPosVel/Target Position and Velocity - GPS corrupted/LOS Calculations/W from body to eci  ==
  q_eci2body : Inport
  Wsat_b : Inport  Port=2
  Quaternion Inverse : aerolibutil/Quaternion Inverse
  Quaternion Rotation : aerolibutil/Quaternion Rotation
  Wsat_eci : Outport
  wires:
  Quaternion Rotation/1 -> Wsat_eci/1
  Wsat_b/1 -> Quaternion Rotation/2
  q_eci2body/1 -> Quaternion Inverse/1
  Quaternion Inverse/1 -> Quaternion Rotation/1

== system TargetPosVel/Target Position and Velocity - GPS corrupted/Pixel shift/UV calculation ==
  Vim_body : Inport
  rho : Inport  Port=2
  True shift : Subsystem
  u_real : Outport
  v_real : Outport  Port=2
  wires:
  rho/1 -> True shift/2(rho)
  Vim_body/1 -> True shift/1(Vim_body)
  True shift/2(v) -> v_real/1
  True shift/1(u) -> u_real/1

== system TargetPosVel/Target Position and Velocity - GPS corrupted/Pixel shift/Vim_body ==
  q : Inport
  vec : Inport  Port=2
  Quaternion Rotation : aerolibutil/Quaternion Rotation
  vec_rot : Outport
  wires:
  Quaternion Rotation/1 -> vec_rot/1
  vec/1 -> Quaternion Rotation/2
  q/1 -> Quaternion Rotation/1

== system TargetPosVel/Target Position and Velocity - GPS corrupted/Pixel shift/Vim_eci ==
  Rtar_eci : Inport
  Vtar_eci : Inport  Port=2
  We_eci : Inport  Port=3
  Cross Product : matrix_library/Cross Product
  Subtract : Sum  Inputs=+-
  Vim_eci : Outport
  wires:
  Vtar_eci/1 -> Subtract/1
  Subtract/1 -> Vim_eci/1
  Cross Product/1 -> Subtract/2
  Rtar_eci/1 -> Cross Product/2
  We_eci/1 -> Cross Product/1

== system TargetPosVel/Target Position and Velocity - Ideal World/LOS Calculations/LOS_hat_eci ==
  Q_eci2body : Inport
  Constant : Constant  Value=pointing_body
  Quaternion Inverse : aerolibutil/Quaternion Inverse
  Quaternion Rotation : aerolibutil/Quaternion Rotation
  LOS_hat_eci : Outport
  wires:
  Q_eci2body/1 -> Quaternion Inverse/1
  Quaternion Inverse/1 -> Quaternion Rotation/1  "q_body2eci"
  Constant/1 -> Quaternion Rotation/2
  Quaternion Rotation/1 -> LOS_hat_eci/1  "LOS_hat_eci"

== system TargetPosVel/Target Position and Velocity - Ideal World/LOS Calculations/W from body to eci  ==
  q_eci2body : Inport
  Wsat_b : Inport  Port=2
  Quaternion Inverse : aerolibutil/Quaternion Inverse
  Quaternion Rotation : aerolibutil/Quaternion Rotation
  Wsat_eci : Outport
  wires:
  Quaternion Inverse/1 -> Quaternion Rotation/1
  q_eci2body/1 -> Quaternion Inverse/1
  Wsat_b/1 -> Quaternion Rotation/2
  Quaternion Rotation/1 -> Wsat_eci/1

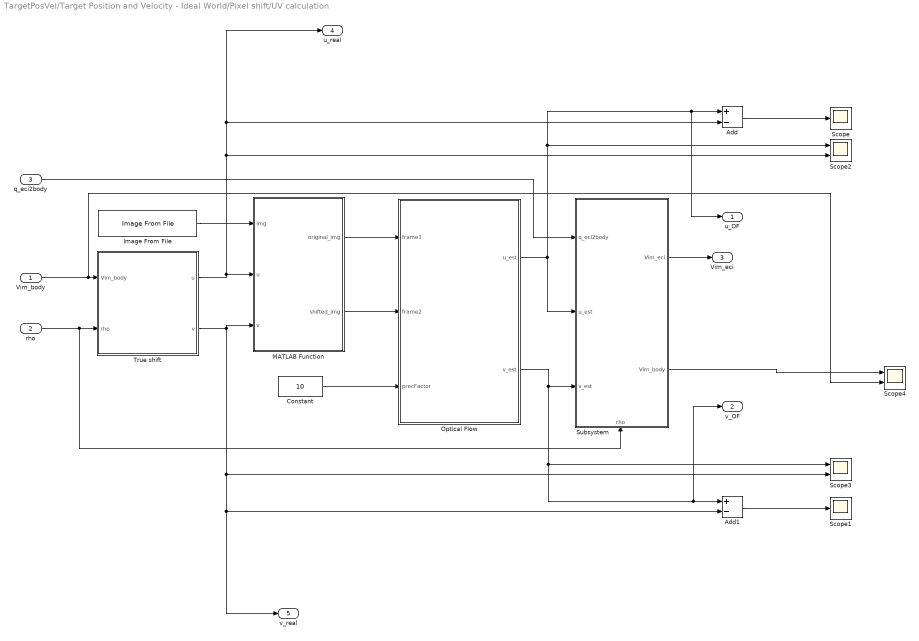
== system TargetPosVel/Target Position and Velocity - Ideal World/Pixel shift/UV calculation ==
  Vim_body : Inport
  rho : Inport  Port=2
  q_eci2body : Inport  Port=3
  Add : Sum  Inputs=+-
  Add1 : Sum  Inputs=+-
  Constant : Constant  Value=10
  Image From File : visionsources/Image From File  Tag=vipblks_nd  FileName=frame.jpg  Ts=inf  imagePorts=One multidimensional signal  OutPortLabels=R|G|B  ImageDataType=Inherit from input image  sdImageDataType=uint(8)  Signed=on  WordLength=16  FractionLengthMode=User-defined  FractionLength=15
  MATLAB Function : MATLAB Function  TreatAsAtomicUnit=on
  Optical Flow : MATLAB Function  TreatAsAtomicUnit=on
  Scope : Scope
      settings: Title=b_u  ActiveDisplayYMinimum=-0.079232845104481253  ActiveDisplayYMaximum=0.13207919106866894
  Scope1 : Scope
      settings: Title=b_v  ActiveDisplayYMinimum=-0.070013971574010736  ActiveDisplayYMaximum=0.11209756833780884  DataLoggingVariableName=ScopeData3
  Scope2 : Scope  NumInputPorts=2
      settings: Title=u vs u_est  ActiveDisplayYMinimum=-32.563714050832083  ActiveDisplayYMaximum=-30.048476216574212
  Scope3 : Scope  NumInputPorts=2
      settings: Title=v vs v_est  ActiveDisplayYMinimum=1.7373438554253244  ActiveDisplayYMaximum=2.0291840160638528  DataLoggingVariableName=ScopeData2
  Scope4 : Scope  NumInputPorts=2
      settings: ActiveDisplayYMinimum=-1  ActiveDisplayYMaximum=1  DataLoggingVariableName=ScopeData6
  Subsystem : Subsystem
      settings: PortSchema="{\"entries\":[{\"content\":{\"sides\":[{\"content\":{\"connectorIds\":[\"In1\",\"In2\",\"In3\"]},\"type\":\"ConnectorPlacement.EquallySpacedRectSide\",\"uuid\":\"00ab2d78-b092-482a-93cf-ae19a1715d5e\"},{\"content\":{\"connectorIds\":[\"Out1\",\"Out2\"],\"side\":\"RIGHT\"},\"type\":\"ConnectorPlacement.EquallySpacedRectSide\",\"uuid\":\"61835ddc-2b31-4e43-8d4a-874cf6b152c0\"},{\"content\":{\"side\":\"TOP\"},\"type\":\"ConnectorPlacement.EquallySpacedRectSide\",\"uuid\":\"ce3dab25-97d8-4e4a-ae1c-056d1a385cfa\"},{\"content\":{\"connectorIds\":[\"In4\"],\"side\":\"BOTTOM\"},\"type\":\"ConnectorPlacement.EquallySpacedRectSide\",\"uuid\":\"e6fea004-ef46-4574-a436-b358c8a4bf67\"}]},\"type\":\"ConnectorPlacement.EquallySpacedConnector\",\"uuid\":\"2a9f85b3-ed2e-41d9-a82c-654d9069fc6b\"}],\"packageUris\":[\"http://schema.mathworks.com/mf0/Connector/R2020b\"],\"version\":\"1.0\"}"
  True shift : Subsystem
  u_OF : Outport
  v_OF : Outport  Port=2
  Vim_eci : Outport  Port=3
  u_real : Outport  Port=4
  v_real : Outport  Port=5
  wires:
  MATLAB Function/1(original_img) -> Optical Flow/1(frame1)
  MATLAB Function/2(shifted_img) -> Optical Flow/2(frame2)
  Image From File/1 -> MATLAB Function/1(img)
  Optical Flow/1(u_est) -> Scope2/1, Add/1, u_OF/1, Subsystem/2(u_est)
  Optical Flow/2(v_est) -> Scope3/1, Add1/1, v_OF/1, Subsystem/3(v_est)
  Constant/1 -> Optical Flow/3(precFactor)
  Vim_body/1 -> Scope4/2, True shift/1(Vim_body)
  rho/1 -> True shift/2(rho), Subsystem/4(rho)
  True shift/1(u) -> u_real/1, Add/2, Scope2/2, MATLAB Function/2(u)
  True shift/2(v) -> MATLAB Function/3(v), Scope3/2, Add1/2, v_real/1
  Add/1 -> Scope/1
  Add1/1 -> Scope1/1
  q_eci2body/1 -> Subsystem/1(q_eci2body)
  Subsystem/1(Vim_eci) -> Vim_eci/1
  Subsystem/2(Vim_body) -> Scope4/1

== system TargetPosVel/Target Position and Velocity - Ideal World/Pixel shift/Vim_body ==
  q : Inport
  vec : Inport  Port=2
  Quaternion Rotation : aerolibutil/Quaternion Rotation
  vec_rot : Outport
  wires:
  q/1 -> Quaternion Rotation/1
  vec/1 -> Quaternion Rotation/2
  Quaternion Rotation/1 -> vec_rot/1

== system TargetPosVel/Target Position and Velocity - Ideal World/Pixel shift/Vim_eci ==
  Rtar_eci : Inport
  Vtar_eci : Inport  Port=2
  We_eci : Inport  Port=3
  Cross Product : matrix_library/Cross Product
  Subtract : Sum  Inputs=+-
  Vim_eci : Outport
  wires:
  We_eci/1 -> Cross Product/1
  Rtar_eci/1 -> Cross Product/2
  Cross Product/1 -> Subtract/2
  Subtract/1 -> Vim_eci/1
  Vtar_eci/1 -> Subtract/1

== system TargetPosVel/Estimation Filter/EKF_rho/Pixel shift/UV calculation ==
  Vim_body : Inport
  rho : Inport  Port=2
  True shift : Subsystem
  u_real : Outport
  v_real : Outport  Port=2
  wires:
  rho/1 -> True shift/2(rho)
  Vim_body/1 -> True shift/1(Vim_body)
  True shift/2(v) -> v_real/1
  True shift/1(u) -> u_real/1

== system TargetPosVel/Estimation Filter/EKF_rho/Pixel shift/Vim_body ==
  q : Inport
  vec : Inport  Port=2
  Quaternion Rotation : aerolibutil/Quaternion Rotation
  vec_rot : Outport
  wires:
  Quaternion Rotation/1 -> vec_rot/1
  vec/1 -> Quaternion Rotation/2
  q/1 -> Quaternion Rotation/1

== system TargetPosVel/Estimation Filter/EKF_rho/Pixel shift/Vim_eci ==
  Rtar_eci : Inport
  Vtar_eci : Inport  Port=2
  We_eci : Inport  Port=3
  Cross Product : matrix_library/Cross Product
  Subtract : Sum  Inputs=+-
  Vim_eci : Outport
  wires:
  Vtar_eci/1 -> Subtract/1
  Subtract/1 -> Vim_eci/1
  Cross Product/1 -> Subtract/2
  Rtar_eci/1 -> Cross Product/2
  We_eci/1 -> Cross Product/1

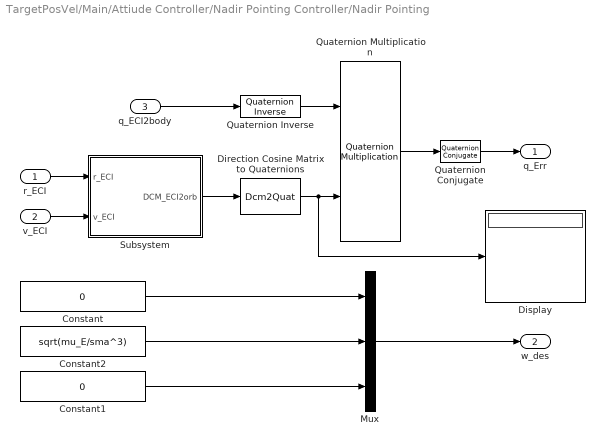
== system TargetPosVel/Main/Attiude Controller/Nadir Pointing Controller/Nadir Pointing ==
  r_ECI : Inport
  v_ECI : Inport  Port=2
  q_ECI2body : Inport  Port=3
  Constant : Constant  Value=0
  Constant1 : Constant  Value=0
  Constant2 : Constant  Value=sqrt(mu_E/sma^3)
  Direction Cosine Matrix to Quaternions : Dcm2Quat
  Display : Display
  Mux : Mux  Inputs=3
  Quaternion Conjugate : aerolibutil/Quaternion Conjugate
  Quaternion Inverse : aerolibutil/Quaternion Inverse
  Quaternion Multiplication : aerolibutil/Quaternion Multiplication
  Subsystem : Subsystem
  q_Err : Outport
  w_des : Outport  Port=2
  wires:
  Quaternion Multiplication/1 -> Quaternion Conjugate/1
  q_ECI2body/1 -> Quaternion Inverse/1
  Constant2/1 -> Mux/2
  Constant1/1 -> Mux/3
  Constant/1 -> Mux/1
  Mux/1 -> w_des/1
  Quaternion Inverse/1 -> Quaternion Multiplication/1
  Direction Cosine Matrix to Quaternions/1 -> Display/1, Quaternion Multiplication/2
  Quaternion Conjugate/1 -> q_Err/1
  v_ECI/1 -> Subsystem/2(v_ECI)
  Subsystem/1(DCM_ECI2orb) -> Direction Cosine Matrix to Quaternions/1
  r_ECI/1 -> Subsystem/1(r_ECI)

== system TargetPosVel/Main/Attiude Controller/Nadir Pointing Controller/Nadir pointing ==
  qErr : Inport
  omega_b : Inport  Port=2
  omega_des_b : Inport  Port=3
  Add2 : Sum  Inputs=+-
  Gain2 : Gain  Gain=kq
  Gain3 : Gain  Gain=kd
  Product1 : Product
  Selector3 : Selector  InputPortWidth=4  IndexOptions=Index vector (dialog)  Indices=[2 3 4]  OutputSizes=1
  Selector4 : Selector  InputPortWidth=4  IndexOptions=Index vector (dialog)  Indices=[1]  OutputSizes=1
  Sum2 : Sum
  g : Outport
  wires:
  Gain3/1 -> Sum2/2
  Gain2/1 -> Product1/2
  Add2/1 -> Gain3/1
  Selector4/1 -> Product1/1
  qErr/1 -> Selector3/1, Selector4/1
  Selector3/1 -> Gain2/1
  omega_des_b/1 -> Add2/2
  Sum2/1 -> g/1
  Product1/1 -> Sum2/1
  omega_b/1 -> Add2/1

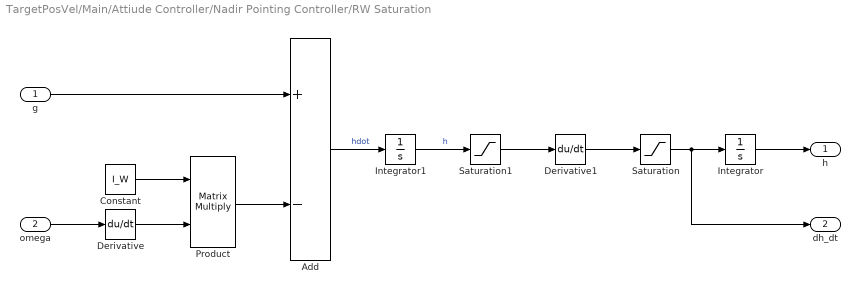
== system TargetPosVel/Main/Attiude Controller/Nadir Pointing Controller/RW Saturation ==
  g : Inport
  omega : Inport  Port=2
  Add : Sum  Inputs=+-
  Constant : Constant  Value=I_W
  Derivative : Derivative
  Derivative1 : Derivative
  Integrator : Integrator  InitialCondition=zeros(3,1)
  Integrator1 : Integrator  InitialCondition=zeros(3,1)
  Product : Product  Multiplication=Matrix(*)
  Saturation : Saturate  UpperLimit=[max_t;max_t;max_t]  LowerLimit=-[max_t;max_t;max_t]
  Saturation1 : Saturate  UpperLimit=[max_h;max_h;max_h]  LowerLimit=-[max_h;max_h;max_h]
  h : Outport
  dh_dt : Outport  Port=2
  wires:
  omega/1 -> Derivative/1
  Constant/1 -> Product/1
  g/1 -> Add/1
  Product/1 -> Add/2
  Derivative/1 -> Product/2
  Integrator/1 -> h/1
  Derivative1/1 -> Saturation/1
  Integrator1/1 -> Saturation1/1  "h"
  Saturation1/1 -> Derivative1/1
  Saturation/1 -> Integrator/1, dh_dt/1
  Add/1 -> Integrator1/1  "hdot"

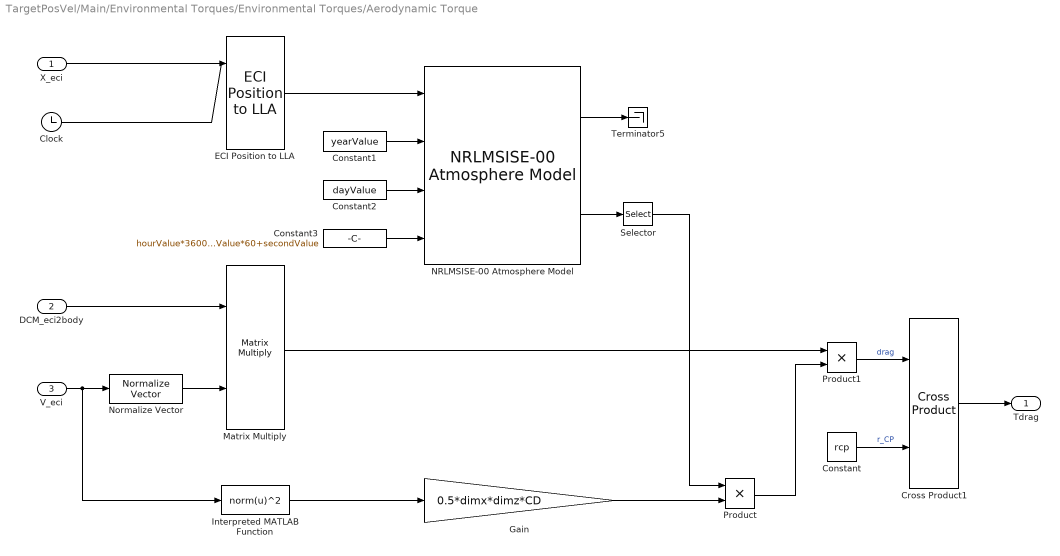
== system TargetPosVel/Main/Environmental Torques/Environmental Torques/Aerodynamic Torque   ==
  X_eci : Inport
  DCM_eci2body : Inport  Port=2
  V_eci : Inport  Port=3
  Clock : Clock
  Constant : Constant  Value=rcp
  Constant1 : Constant  Value=yearValue
  Constant2 : Constant  Value=dayValue
  Constant3 : Constant  Value=hourValue*3600+minuteValue*60+secondValue
  Cross Product1 : matrix_library/Cross Product
  ECI Position to LLA : aerolibtransform2/ECI Position to LLA  red=IAU-2000/2006  year=yearValue  month=January  day=1  hour=hourValue  min=minuteValue  sec=secondValue  deltaT=Sec  errorflag=Warning  extraparamflag=off  eunits=Metric (MKS)  earthmodel=WGS84  flat=1/298.257223563  eqradius=6378137
      settings: AttributesFormatString=%<red>
  Gain : Gain  Gain=0.5*dimx*dimz*CD
  Interpreted MATLAB Function : MATLABFcn  MATLABFcn=norm(u)^2
  Matrix Multiply : Product  Multiplication=Matrix(*)
  NRLMSISE-00 Atmosphere Model : aerolibatmos2/NRLMSISE-00 Atmosphere Model  units=Metric (MKS)  lst_input=off  flux_ap_input=off  flags_input=Internal  flags=ones(1,23)  oxygen_in=off  action=None
  Normalize Vector : vrlib/Utilities/Normalize Vector  maxzero=0
  Product : Product
  Product1 : Product
  Selector : Selector  InputPortWidth=9  IndexOptions=Index vector (dialog)  Indices=6  OutputSizes=1
  Terminator5 : Terminator
  Tdrag : Outport
  wires:
  X_eci/1 -> ECI Position to LLA/1
  Gain/1 -> Product/2
  V_eci/1 -> Interpreted MATLAB Function/1, Normalize Vector/1
  Interpreted MATLAB Function/1 -> Gain/1
  DCM_eci2body/1 -> Matrix Multiply/1
  Normalize Vector/1 -> Matrix Multiply/2
  Matrix Multiply/1 -> Product1/1
  Product/1 -> Product1/2
  Cross Product1/1 -> Tdrag/1
  Clock/1 -> ?
  Product1/1 -> Cross Product1/1  "drag"
  Constant/1 -> Cross Product1/2  "r_CP"
  Constant1/1 -> NRLMSISE-00 Atmosphere Model/2
  Constant3/1 -> NRLMSISE-00 Atmosphere Model/4
  ECI Position to LLA/1 -> NRLMSISE-00 Atmosphere Model/1
  Constant2/1 -> NRLMSISE-00 Atmosphere Model/3
  NRLMSISE-00 Atmosphere Model/2 -> Selector/1
  NRLMSISE-00 Atmosphere Model/1 -> Terminator5/1
  Selector/1 -> Product/1

== system TargetPosVel/Main/Environmental Torques/Environmental Torques/Gravity Gradient Torque ==
  DCM_eci2body : Inport
  X_eci : Inport  Port=2
  Constant : Constant  Value=I
  Cross Product : matrix_library/Cross Product
  Divide : Product  Inputs=*/
  Gain : Gain  Gain=3*mu_E
  Interpreted MATLAB Function : MATLABFcn  MATLABFcn=norm(u)^3
  Matrix Multiply : Product  Multiplication=Matrix(*)
  Matrix Multiply2 : Product  Multiplication=Matrix(*)
  Normalize Vector1 : vrlib/Utilities/Normalize Vector  maxzero=0
  Tgg : Outport
  wires:
  X_eci/1 -> Interpreted MATLAB Function/1, Matrix Multiply/2
  Normalize Vector1/1 -> Matrix Multiply2/2, Cross Product/1
  Divide/1 -> Tgg/1
  Matrix Multiply/1 -> Normalize Vector1/1
  Gain/1 -> Divide/1
  Matrix Multiply2/1 -> Cross Product/2
  Constant/1 -> Matrix Multiply2/1
  DCM_eci2body/1 -> Matrix Multiply/1
  Interpreted MATLAB Function/1 -> Divide/2  "Rs^3"
  Cross Product/1 -> Gain/1

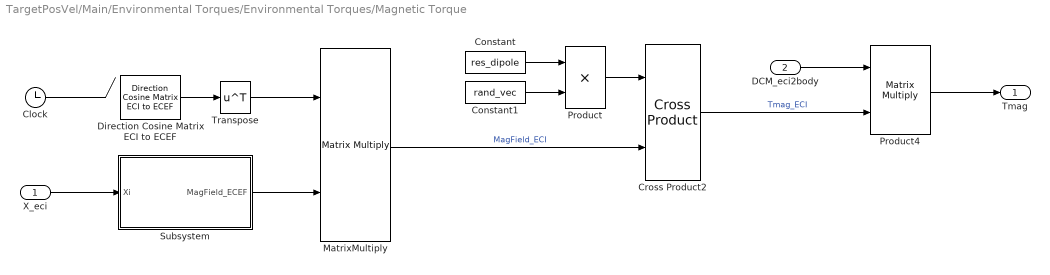
== system TargetPosVel/Main/Environmental Torques/Environmental Torques/Magnetic Torque ==
  X_eci : Inport
  DCM_eci2body : Inport  Port=2
  Clock : Clock
  Constant : Constant  Value=res_dipole
  Constant1 : Constant  Value=rand_vec
  Cross Product2 : matrix_library/Cross Product
  Direction Cosine Matrix ECI to ECEF : aerolibtransform2/Direction Cosine Matrix ECI to ECEF  red=IAU-2000/2006  year=yearValue  month=January  day=1  hour=hourValue  min=minuteValue  sec=secondValue  deltaT=Sec  errorflag=Error  extraparamflag=off
      settings: AttributesFormatString=%<red>
  MatrixMultiply : Product  Multiplication=Matrix(*)
  Product : Product
  Product4 : Product  Multiplication=Matrix(*)
  Subsystem : Subsystem
  Transpose : Math  Operator=transpose
  Tmag : Outport
  wires:
  Product4/1 -> Tmag/1
  Constant/1 -> Product/1
  Product/1 -> Cross Product2/1
  DCM_eci2body/1 -> Product4/1
  Constant1/1 -> Product/2
  MatrixMultiply/1 -> Cross Product2/2  "MagField_ECI"
  Cross Product2/1 -> Product4/2  "Tmag_ECI"
  X_eci/1 -> Subsystem/1(Xi)
  Subsystem/1(MagField_ECEF) -> MatrixMultiply/2
  Clock/1 -> ?
  Transpose/1 -> MatrixMultiply/1
  Direction Cosine Matrix ECI to ECEF/1 -> Transpose/1

== system TargetPosVel/Main/Environmental Torques/Environmental Torques/Solar Radiation Pressure Torque ==
  DCM_eci2body : Inport
  X_eci : Inport  Port=2
  t_JD : Inport  Port=3
  Add2 : Sum  Inputs=-+
  Constant : Constant  Value=rcp
  Cross Product3 : matrix_library/Cross Product
  Gain3 : Gain  Gain=-Phi*dimx*dimz*(1+q)/c
  Matrix Multiply4 : Product  Multiplication=Matrix(*)
  Normalize Vector2 : vrlib/Utilities/Normalize Vector  maxzero=0
  Planetary Ephemeris : PlanetaryEphem  units=m,m/s  target=Sun  outputVelocity=off
  T_srp : Outport
  wires:
  Gain3/1 -> Cross Product3/2
  Add2/1 -> Normalize Vector2/1
  Normalize Vector2/1 -> Matrix Multiply4/2
  Matrix Multiply4/1 -> Gain3/1
  X_eci/1 -> Add2/1
  t_JD/1 -> Planetary Ephemeris/1
  Cross Product3/1 -> T_srp/1
  Constant/1 -> Cross Product3/1
  DCM_eci2body/1 -> Matrix Multiply4/1
  Planetary Ephemeris/1 -> Add2/2  "Xi_SUN"

== system TargetPosVel/Main/Spacecraft Dynamics/GPS/NED to ECI ==
  LLA : Inport
  V_NED : Inport  Port=2
  Reci2ned : Inport  Port=3
  LLA to ECI Position : aerolibtransform2/LLA to ECI Position  red=IAU-2000/2006  year=yearValue  month=January  day=1  hour=hourValue  min=minuteValue  sec=secondValue  deltaT=Sec  errorflag=Error  extraparamflag=off  eunits=Metric (MKS)  earthmodel=WGS84  flat=1/298.257223563  eqradius=6378137
      settings: AttributesFormatString=%<red>
  MatrixMultiply : Product  Multiplication=Matrix(*)
  Transpose2 : Math  Operator=transpose
  Transpose3 : Math  Operator=transpose
  X_GPS : Outport
  V_GPS : Outport  Port=2
  wires:
  Transpose2/1 -> MatrixMultiply/1
  V_NED/1 -> Transpose3/1
  Reci2ned/1 -> Transpose2/1
  LLA/1 -> LLA to ECI Position/1
  Transpose3/1 -> MatrixMultiply/2
  LLA to ECI Position/1 -> X_GPS/1
  MatrixMultiply/1 -> V_GPS/1
  [time] -> LLA to ECI Position/2

== system TargetPosVel/Main/Spacecraft Dynamics/GPS/V from ECI to NED ==
  Xi : Inport
  Vi : Inport  Port=2
  MATLAB Function1 : MATLAB Function  TreatAsAtomicUnit=on
  Product2 : Product  Multiplication=Matrix(*)
  Vned : Outport
  Reci2ned : Outport  Port=2
  wires:
  Xi/1 -> MATLAB Function1/1(X_icrf)
  MATLAB Function1/1(Reci2ned) -> Reci2ned/1, Product2/1
  Vi/1 -> Product2/2
  Product2/1 -> Vned/1

== system TargetPosVel/Target Position and Velocity - GPS corrupted/Pixel shift/UV calculation/True shift ==
  Vim_body : Inport
  rho : Inport  Port=2
  Demux1 : Demux  Outputs=2
  Divide1 : Product  Inputs=*/
  Gain3 : Gain  Gain=K_optics
  u : Outport
  v : Outport  Port=2
  wires:
  Demux1/1 -> u/1
  rho/1 -> Divide1/2
  Vim_body/1 -> Gain3/1
  Gain3/1 -> Divide1/1
  Divide1/1 -> Demux1/1
  Demux1/2 -> v/1

== system TargetPosVel/Target Position and Velocity - Ideal World/Pixel shift/UV calculation/Subsystem ==
  q_eci2body : Inport
  u_est : Inport  Port=2
  v_est : Inport  Port=3
  rho : Inport  Port=4
  Gain : Gain  Gain=1/K_optics
  Mux : Mux  Inputs=3
  Product : Product
  Quaternion Inverse : aerolibutil/Quaternion Inverse
  Quaternion Rotation : aerolibutil/Quaternion Rotation
  Zero : Constant  Value=0  OutDataTypeStr=Inherit: Inherit via back propagation
  Vim_eci : Outport
  Vim_body : Outport  Port=2
  wires:
  u_est/1 -> Mux/1
  v_est/1 -> Mux/2
  Zero/1 -> Mux/3
  q_eci2body/1 -> Quaternion Inverse/1
  rho/1 -> Gain/1
  Gain/1 -> Product/2
  Mux/1 -> Product/1
  Product/1 -> Vim_body/1, Quaternion Rotation/2  "Vim_body"
  Quaternion Inverse/1 -> Quaternion Rotation/1  "q_body2eci"
  Quaternion Rotation/1 -> Vim_eci/1

== system TargetPosVel/Target Position and Velocity - Ideal World/Pixel shift/UV calculation/True shift ==
  Vim_body : Inport
  rho : Inport  Port=2
  Demux1 : Demux  Outputs=2
  Divide1 : Product  Inputs=*/
  Gain3 : Gain  Gain=K_optics
  u : Outport
  v : Outport  Port=2
  wires:
  Demux1/2 -> v/1
  Divide1/1 -> Demux1/1
  Gain3/1 -> Divide1/1
  Vim_body/1 -> Gain3/1
  rho/1 -> Divide1/2
  Demux1/1 -> u/1

== system TargetPosVel/Estimation Filter/EKF_rho/Pixel shift/UV calculation/True shift ==
  Vim_body : Inport
  rho : Inport  Port=2
  Demux1 : Demux  Outputs=2
  Divide1 : Product  Inputs=*/
  Gain3 : Gain  Gain=K_optics
  u : Outport
  v : Outport  Port=2
  wires:
  Demux1/1 -> u/1
  rho/1 -> Divide1/2
  Vim_body/1 -> Gain3/1
  Gain3/1 -> Divide1/1
  Divide1/1 -> Demux1/1
  Demux1/2 -> v/1
